simulink model "Sim_ANN"  (R2014a)
settings: Solver=ode45  StartTime=0.0  StopTime=10.0  RelTol=1e-3
settings Model: Creator=johan  LastModifiedBy=johan

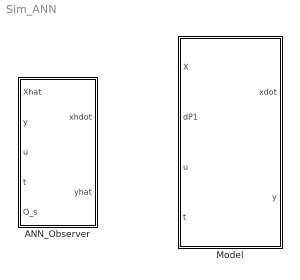
== system Sim_ANN ==
  ANN_Observer : MATLAB Function  TreatAsAtomicUnit=on
  Model : MATLAB Function  TreatAsAtomicUnit=on

== matlab function Sim_ANN/ANN_Observer ==
  data: Xhat input; y input; u input; xhdot output; yhat output; t input; O_s input
function [xhdot, yhat] = fcn(Xhat,y,u,t,O_s)
    
    Xhat = [x1 x2 x3 x4 x5 x6 x7 x8 x9 x10]';
    
    J1 = 10;
    omg1 = 0.05;
    mu1 = 1.5;
    Tg1 = 0.12;
    Ttu1 = 0.2;
    T12 = 0.198;
    % R = 10*eye(2); %%%%%%%
    Beta1 = 21.5;
    
    J2 = 10;
    omg2 = 0.05;
    mu2 = 1;
    Tg2 = 0.18;
    Ttu2 = 0.45;
    T21 = 0.198;
    % Q = 10*eye(2); %%%%%%%%%
    Beta2 = 21;
    
    
    A11 = [-mu1/J1 1/J1 0 -1/J1 0
        0 -1/Ttu1 1/Ttu1 0 0
        -1/(omg1*Tg1) 0 -1/Tg1 0 0
        2*pi*(T12 + T21) 0 0 0 0
        Beta1 0 0 1 0];
   
    A22 = [-mu2/J2 1/J2 0 -1/J2 0
        0 -1/Ttu2 1/Ttu2 0 0
        -1/(omg2*Tg2) 0 -1/Tg2 0 0
        2*pi*(T12 + T21) 0 0 0 0
        Beta2 0 0 1 0];
    A12 = [0 0 0 0 0
        0 0 0 0 0
        0 0 0 0 0
        -2*pi*T12 0 0 0 0
        0 0 0 0 0];
        
    A21 = [0 0 0 0 0
        0 0 0 0 0
        0 0 0 0 0
        -2*pi*T21 0 0 0 0
        0 0 0 0 0];
        
    A = [A11 A12; A21 A22];
    
    B1 = [0 0 1/Tg1 0 0]';
    B2 = [0 0 1/Tg2 0 0]';
    B = diag([B1' B2']');
    
%     D1 = [-1/J1 0 0 0 0]';
%     D2 = [-1/J2 0 0 0 0]';
     
    L = 1;%%%%%
    O_s = zeros(10,1);
    Tao = 0.01;
    
    for i = 1:10
        Zi = 
        Sigma_z = 1-exp(Zi)/1+exp(Zi);
        O_s(i) = W(i)*Sigma_z;
    end
    
    
    O_s = Wi*Sigma_z;
    
    %dP1 = 1; %%%%%%%%%%%%%%%%%%
    xhdot = A*Xhat + B*u + L*(y - yhat);
    yhat = C*Xhat + O_s;
end

== matlab function Sim_ANN/Model ==
  data: X input; dP1 input; u input; xdot output; t input; y output
function [xdot, y] = fcn(X,dP1,u,t)
    
    X = [x1 x2 x3 x4 x5 x6 x7 x8 x9 x10]';
    
    J1 = 10;
    omg1 = 0.05;
    mu1 = 1.5;
    Tg1 = 0.12;
    Ttu1 = 0.2;
    T12 = 0.198;
    % R = 10*eye(2); %%%%%%%
    Beta1 = 21.5;
    
    J2 = 10;
    omg2 = 0.05;
    mu2 = 1;
    Tg2 = 0.18;
    Ttu2 = 0.45;
    T21 = 0.198;
    % Q = 10*eye(2); %%%%%%%%%
    Beta2 = 21;
    
    
    A11 = [-mu1/J1 1/J1 0 -1/J1 0
        0 -1/Ttu1 1/Ttu1 0 0
        -1/(omg1*Tg1) 0 -1/Tg1 0 0
        2*pi*(T12 + T21) 0 0 0 0
        Beta1 0 0 1 0];
   
    A22 = [-mu2/J2 1/J2 0 -1/J2 0
        0 -1/Ttu2 1/Ttu2 0 0
        -1/(omg2*Tg2) 0 -1/Tg2 0 0
        2*pi*(T12 + T21) 0 0 0 0
        Beta2 0 0 1 0];
    A12 = [0 0 0 0 0
        0 0 0 0 0
        0 0 0 0 0
        -2*pi*T12 0 0 0 0
        0 0 0 0 0];
        
    A21 = [0 0 0 0 0
        0 0 0 0 0
        0 0 0 0 0
        -2*pi*T21 0 0 0 0
        0 0 0 0 0];
        
    A = [A11 A12; A21 A22];
    
    B1 = [0 0 1/Tg1 0 0]';
    B2 = [0 0 1/Tg2 0 0]';
    B = diag([B1' B2']');
    
    D1 = [-1/J1 0 0 0 0]';
    D2 = [-1/J2 0 0 0 0]';
    
    D = diag([D1' D2']');
    C = eye(2);
    %dP1 = 1; %%%%%%%%%%%%%%%%%%
    xdot = A*x + B*u + D*dPl;
    y = C*xdot + d;
end
